simulink model "lec11_slides_ex4"  (R2023b)
settings: Solver=VariableStepAuto  StartTime=0.0  StopTime=1  RelTol=1e-3
settings Model: Creator=john  LastModifiedBy=john

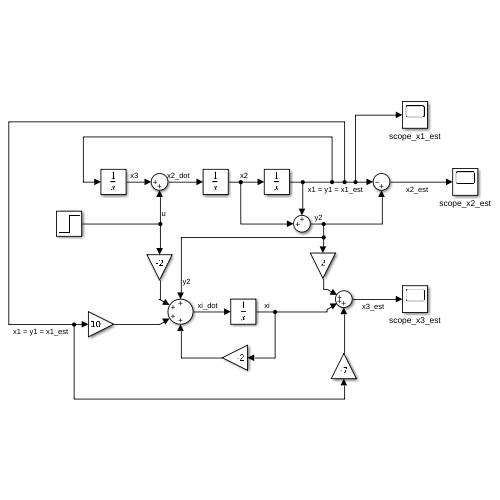
[thumbnail: Simulink's stored preview of the top-level diagram]
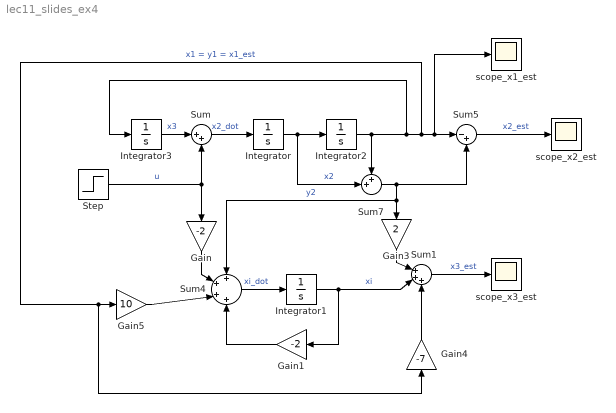
== system lec11_slides_ex4 ==
  Gain : Gain  Gain=-2
  Gain1 : Gain  Gain=-2
  Gain3 : Gain  Gain=2
  Gain4 : Gain  Gain=-7
  Gain5 : Gain  Gain=10
  Integrator{,1..3} (4 alike) : Integrator
  Step : Step  Time=0  SampleTime=0
  Sum : Sum  Inputs=|++
  Sum1 : Sum  Inputs=|+++
  Sum4 : Sum  Inputs=++++
  Sum5 : Sum  Inputs=|-+
  Sum7 : Sum  Inputs=++|
  scope_x1_est : Scope
  scope_x2_est : Scope
  scope_x3_est : Scope
  wires:
  Gain/1 -> Sum4/2
  Sum/1 -> Integrator/1  "x2_dot"
  Step/1 -> Sum/2, Gain/1  "u"
  Sum4/1 -> Integrator1/1  "xi_dot"
  Integrator1/1 -> Gain1/1, Sum1/2  "xi"
  Integrator/1 -> Sum7/2, Integrator2/1  "x2"
  Integrator2/1 -> Integrator3/1, Sum5/1, scope_x1_est/1, Gain4/1, Gain5/1, Sum7/1  "x1 = y1 = x1_est"
  Integrator3/1 -> Sum/1  "x3"
  Sum7/1 -> Sum4/1, Gain3/1, Sum5/2  "y2"
  Sum5/1 -> scope_x2_est/1  "x2_est"
  Gain3/1 -> Sum1/1
  Gain4/1 -> Sum1/3
  Gain5/1 -> Sum4/3
  Gain1/1 -> Sum4/4
  Sum1/1 -> scope_x3_est/1  "x3_est"
